simulink model "Quad_PID_FUSION_Close_Loop"  (R2023b)
settings: Solver=ode1  StartTime=0.0  StopTime=400  FixedStep=0.01  RelTol=1e-3
values from neighbouring files (symbols this model uses):
  Quad_Model = struct(     'Ixx', 0.016,      'Iyy', 0.016,      'Izz', 0.0274,      'Im', 3.789e-6,      'mass', 1,      'g', 9.8)    [Quad_PID_FUSION_Pipeline.m]    (also in Quad_PID_FUSION_Pipeline_Close_Loop_Attack.m; Quad_PID_FUSION_Pipeline_Close_Loop_Attack_Pipeline.m; Quad_PID_FUSION_Pipeline_Close_Loop_Attack_Pipeline_Reach.m; Quad_PID_FUSION_Pipeline_Close_Loop_Attack_Pipeline_Repeat_V5.m)
  s_x_0 = 0.0    (= 0)    [Quad_PID_FUSION_Pipeline.m]    (also in Quad_PID_FUSION_Pipeline_Loop_Attack_Execution.m = current_norm * cos(angle))
  s_y_0 = 0.0    (= 0)    [Quad_PID_FUSION_Pipeline.m]    (also in Quad_PID_FUSION_Pipeline_Loop_Attack_Execution.m = current_norm * sin(angle))
undefined symbols (not defined in the file or in its folder): DiscIntNeverNeededParam
libraries: simulink x9, rllib x1
(part 1 of 2)
settings Model: SimulationMode=accelerator  Creator=Qi  LastModifiedBy=32977
settings SolverCC: AlgebraicLoopSolver=TrustRegion
settings DataIOCC: ReturnWorkspaceOutputs=off
settings DebuggingCC: UnconnectedInputMsg=warning  UnconnectedOutputMsg=warning  UnconnectedLineMsg=warning  ArithmeticOperatorsInVariantConditions=warning
settings ModelReferenceCC: EnableRefExpFcnMdlSchedulingChecks=on
settings SFSimCC: CustomCodeUndefinedFunction=UseInterfaceOnly

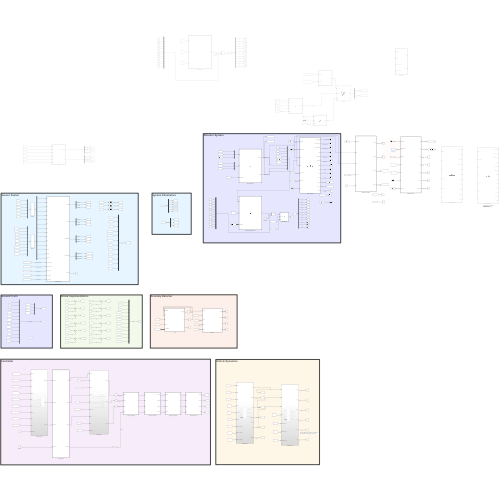
[thumbnail: Simulink's stored preview of the top-level diagram]
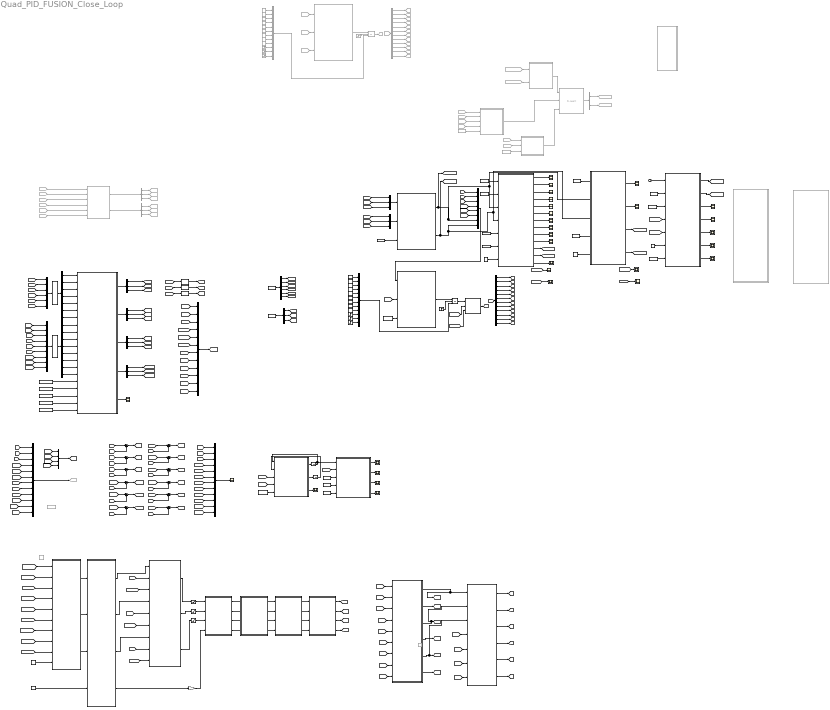
== system Quad_PID_FUSION_Close_Loop ==
  note: Fix the problem of non-covergence at small spoofing distance by adaptive PID tuning
  note: Attacker System
  note: System Parameters
  note: Anomaly Detector
  note: Sensor Fusion
  note: Vehicle Dynamics
  note: Controller
  note: Ground Truth
  note: Attack Implementation
  note: The initial condition of the integrator here is changed to 10,
      | so the intial position of drone is going to be [0,0,10]
  Attack Dynamics : MATLAB Function  Commented=on  TreatAsAtomicUnit=on
  Attack Injection : MATLAB Function  TreatAsAtomicUnit=on
  Attack Time : Step  Time=0  SampleTime=0
  Attacker Observation : MATLAB Function  TreatAsAtomicUnit=on
  Attacker Redirection MPC : MATLAB Function  TreatAsAtomicUnit=on
  Attacker redirection : MATLAB Function  TreatAsAtomicUnit=on
  Attacker redirection1 : MATLAB Function  Commented=on  TreatAsAtomicUnit=on
  Attacker redirection2 : MATLAB Function  Commented=on  TreatAsAtomicUnit=on
  Attacker redirection3 : MATLAB Function  TreatAsAtomicUnit=on
  Attitude Controller : Subsystem
  Attitude Dynamics : Subsystem
  Clock : Clock
  Constant : Constant  Commented=on  Value=10
  Constant{1..2,13..19} (9 alike) : Constant  Value=0
  Constant{4..12} (9 alike) : Constant  Commented=on  Value=0
  Constant20 : Constant  Value=Quad_Model  OutDataTypeStr=Bus: Quad_Model_Bus
  Constant21 : Constant  Value=Quad_Model  OutDataTypeStr=Bus: Quad_Model_Bus
  Constant22 : Constant  Value=0.01
  Constant23 : Constant  Value=0.01
  Constant24 : Constant  Value=0.01
  Constant3 : Constant  Value=0.5
  Demux : Demux  Outputs=9
  Demux1 : Demux  Commented=on  Outputs=3
  Demux{2,4..6,10} (5 alike) : Demux  Outputs=3
  Demux11 : Demux  Outputs=12
  Demux12 : Demux  Commented=on  Outputs=2
  Demux3 : Demux  Commented=on  Outputs=3
  Demux7 : Demux  Commented=on  Outputs=12
  Demux8 : Demux  Outputs=6
  Demux9 : Demux  Outputs=6
  Detector : MATLAB Function  TreatAsAtomicUnit=on
  Discrete Derivative3 : simulink/Discrete/Discrete Derivative  gainval=1.0  ICPrevScaledInput=0.0  OutMin=[]  OutMax=[]  OutDataType=fixdt(1, 16)  OutScaling=2^-10  DoSatur=off
  Discrete Derivative4 : simulink/Discrete/Discrete Derivative  gainval=1.0  ICPrevScaledInput=0.0  OutMin=[]  OutMax=[]  OutDataType=fixdt(1, 16)  OutScaling=2^-10  DoSatur=off
  Discrete Derivative5 : simulink/Discrete/Discrete Derivative  gainval=1.0  ICPrevScaledInput=0.0  OutMin=[]  OutMax=[]  OutDataType=fixdt(1, 16)  OutScaling=2^-10  DoSatur=off
  EKF : MATLAB Function  TreatAsAtomicUnit=on
  From Workspace1 : FromWorkspace  VariableName=System_Noise
  From Workspace10 : FromWorkspace  VariableName=WaypointSeries
  From Workspace11 : FromWorkspace  Commented=on  VariableName=s_x_0_series
  From Workspace12 : FromWorkspace  VariableName=Attacker_Noise
  From Workspace13 : FromWorkspace  VariableName=Spoofing_Target
  From Workspace14 : FromWorkspace  VariableName=S_Norm
  From Workspace15 : FromWorkspace  VariableName=Delta_S_Lim
  From Workspace16 : FromWorkspace  VariableName=Spoofing_Target
  From Workspace17 : FromWorkspace  VariableName=Spoofing_Target
  From Workspace18 : FromWorkspace  VariableName=Delta_S_Lim
  From Workspace19 : FromWorkspace  Commented=on  VariableName=Spoofing_Target
  From Workspace2 : FromWorkspace  VariableName=GPS_Position_Noise
  From Workspace20 : FromWorkspace  Commented=on  VariableName=Spoofing_Target
  From Workspace21 : FromWorkspace  VariableName=Target_R
  From Workspace22 : FromWorkspace  VariableName=Delta_S_Lim
  From Workspace23 : FromWorkspace  VariableName=Attack_Start_T
  From Workspace3 : FromWorkspace  VariableName=GPS_Velocity_Noise
  From Workspace4 : FromWorkspace  VariableName=IMU_Acc_Noise
  From Workspace5 : FromWorkspace  VariableName=IMU_Gyro_Noise
  From Workspace6 : FromWorkspace  VariableName=IMU_Mag_Noise
  From Workspace7 : FromWorkspace  VariableName=Gamma
  From Workspace8 : FromWorkspace  VariableName=Delta_1
  From Workspace9 : FromWorkspace  VariableName=Delta_2
  From102 : From  Commented=on  GotoTag=pos_y_diff
  From103 : From  Commented=on  GotoTag=pos_z_diff
  From142 : From  Commented=on  GotoTag=vel_y
  From143 : From  Commented=on  GotoTag=pos_x
  From144 : From  Commented=on  GotoTag=pos_x
  From145 : From  Commented=on  GotoTag=pos_y
  From146 : From  Commented=on  GotoTag=pos_y
  From147 : From  Commented=on  GotoTag=vel_x
  From150 : From  Commented=on  GotoTag=attacker_pos_obs
  From151 : From  Commented=on  GotoTag=attacker_vel_obs
  From16 : From  Commented=on  GotoTag=pos_x_diff
  From20 : From  Commented=on  GotoTag=vel_y_diff
  From21 : From  Commented=on  GotoTag=vel_z_diff
  From49 : From  Commented=on  GotoTag=input
  From50 : From  Commented=on  GotoTag=X
  From51 : From  Commented=on  GotoTag=s
  From52 : From  Commented=on  GotoTag=s
  From56 : From  Commented=on  GotoTag=vel_x_diff
  GPS : MATLAB Function  Commented=on  TreatAsAtomicUnit=on
  GPS Sensor : MATLAB Function  Commented=on  TreatAsAtomicUnit=on
  GPS Spoofing Attack Dynamics : MATLAB Function  TreatAsAtomicUnit=on
  GPS ZOH : ZeroOrderHold  SampleTime=0.1
  GPSIMUFUSION : MATLAB Function  TreatAsAtomicUnit=on
  Gain1 : Gain  Gain=20
  Goto12 : Goto  Commented=on  GotoTag=pos_x_gps
  Goto13 : Goto  Commented=on  GotoTag=pos_y_gps
  Goto14 : Goto  Commented=on  GotoTag=pos_z_gps
  Goto15 : Goto  Commented=on  GotoTag=vel_x_gps
  Goto16 : Goto  Commented=on  GotoTag=vel_y_gps
  Goto17 : Goto  Commented=on  GotoTag=vel_z_gps
  Goto24 : Goto  Commented=on  GotoTag=s
  Goto25 : Goto  Commented=on  GotoTag=s_1
  Goto26 : Goto  Commented=on  GotoTag=s_2
  Goto27 : Goto  Commented=on  GotoTag=s_3
  Goto28 : Goto  Commented=on  GotoTag=s_4
  Goto41 : Goto  Commented=on  GotoTag=s_5
  Goto42 : Goto  Commented=on  GotoTag=s_6
  Goto43 : Goto  Commented=on  GotoTag=s_7
  Goto44 : Goto  Commented=on  GotoTag=s_8
  Goto45 : Goto  Commented=on  GotoTag=s_9
  Goto46 : Goto  Commented=on  GotoTag=s_10
  Goto47 : Goto  Commented=on  GotoTag=s_11
  Goto48 : Goto  Commented=on  GotoTag=s_12
  Goto54 : Goto  Commented=on  GotoTag=X
  Goto91 : Goto  Commented=on  GotoTag=new_s_vx_rl
  Goto92 : Goto  Commented=on  GotoTag=new_s_vy_rl
  IMU ZOH : ZeroOrderHold  SampleTime=0.01
  Integrator1 : Integrator  InitialCondition=1*[0,0,0,0,0,0,0,0,10,0,0,0]
  Integrator100 : Integrator  Commented=on  ExternalReset=rising  InitialConditionSource=external  InitialCondition=0.002*[1,0,0,0,0,0,0,0,0,0,0,0]
  Integrator2 : Integrator  InitialCondition=0*eye(12)
  Integrator4 : Integrator  ExternalReset=rising  InitialConditionSource=external  InitialCondition=0.002*[1,0,0,0,0,0,0,0,0,0,0,0]
  MATLAB Function : MATLAB Function  Commented=on  TreatAsAtomicUnit=on
  MATLAB Function1 : MATLAB Function  Commented=on  TreatAsAtomicUnit=on
  MATLAB Function2 : MATLAB Function  Commented=on  TreatAsAtomicUnit=on
  Mux : Mux
  Mux{1..2,6..7} (4 alike) : Mux  Inputs=12
  Mux10 : Mux  Inputs=8
  Mux3 : Mux  Inputs=9
  Mux4 : Mux  Inputs=6
  Mux5 : Mux  Commented=on  Inputs=12
  Mux8 : Mux  Inputs=3
  Mux9 : Mux  Inputs=3
  Position Controller : Subsystem
  Position Dynamics : Subsystem
  RLSpoofer : rllib/RL Agent  Commented=on  Agent=agent  ExternalActionAsInput=off  ProvideLastAction=off  ProvideCumRwd=off  TreatAsDirectFeedthrough=on  UseStrictObservationDataTypes=off
  Saturation : Saturate  UpperLimit=1  LowerLimit=-1
  Saturation1 : Saturate  UpperLimit=1  LowerLimit=-1
  Saturation2 : Saturate  UpperLimit=1  LowerLimit=-1
  Scope{,1..28} (29 alike) : Scope
  Step1 : Step  Commented=on  Time=0  After=s_y_0  SampleTime=0
  Step2 : Step  Commented=on  Time=0  After=0  SampleTime=0
  Step3 : Step  Commented=on  Time=3  SampleTime=0
  Step4 : Step  Commented=on  Time=0  After=s_x_0  SampleTime=0
  Step5 : Step  Time=0  After=0  SampleTime=0
  Step6 : Step  Time=0  After=0  SampleTime=0
  Step8 : Step  Time=0  After=0  SampleTime=0
  Sum{12..23} (12 alike) : Sum  Inputs=|+-
  Thrust_to_Attitude : MATLAB Function  TreatAsAtomicUnit=on
  "disturbance " : Constant  Commented=on  Value=0
  "motor_speed_to_throttle " : MATLAB Function  TreatAsAtomicUnit=on
  motor_speed_to_thrust : MATLAB Function  TreatAsAtomicUnit=on
  throttle_to_motor_speed : MATLAB Function  TreatAsAtomicUnit=on
  thrust_to_motor_speed : MATLAB Function  TreatAsAtomicUnit=on
  yaw_sp : Constant  Value=0
  wires:
  yaw_sp/1 -> Thrust_to_Attitude/4(yaw_setpoint)
  Thrust_to_Attitude/4(thrust_body) -> Gain1/1
  [pos_x_fused] -> Position Controller/2(pos_x)
  [target_y] -> Position Controller/4(pos_sp_y)
  [pos_z_fused] -> Position Controller/8(pos_z)
  [target_z] -> Position Controller/7(pos_sp_z)
  Position Controller/1(thrust_sp_x) -> Thrust_to_Attitude/1(thrust_enu_x)
  Position Controller/2(thrust_sp_y) -> Thrust_to_Attitude/2(thrust_enu_y)
  Position Controller/3(thrust_sp_z) -> Thrust_to_Attitude/3(thrust_enu_z)
  [yaw_fused] -> Attitude Controller/8(yaw)
  [roll_fused] -> Attitude Controller/2(roll)
  [pitch_fused] -> Attitude Controller/5(pitch)
  Thrust_to_Attitude/1(roll_sp) -> Attitude Controller/1(roll_sp)
  Thrust_to_Attitude/2(pitch_sp) -> Attitude Controller/4(pitch_sp)
  Thrust_to_Attitude/3(yaw_sp) -> Attitude Controller/7(yaw_sp)
  Attitude Controller/2(torque_y) -> Saturation1/1
  Attitude Controller/1(torque_x) -> Saturation/1
  Attitude Controller/3(torque_z) -> Saturation2/1
  [vel_x_fused] -> Position Controller/3(vel_x)
  [pos_y_fused] -> Position Controller/5(pos_y)
  [vel_y_fused] -> Position Controller/6(vel_y)
  [vel_z_fused] -> Position Controller/9(vel_z)
  [roll_rate_fused] -> Attitude Controller/3(roll_rate)
  [pitch_rate_fused] -> Attitude Controller/6(pitch_rate)
  [yaw_rate_fused] -> Attitude Controller/9(yaw_rate)
  Attitude Dynamics/3(pitch) -> Position Dynamics/2(pitch), [pitch]  "pitch"
  Attitude Dynamics/1(roll) -> [roll], Position Dynamics/1(roll)  "roll"
  Attitude Dynamics/5(yaw) -> [yaw], Position Dynamics/3(yaw)  "yaw"
  [roll_rate] -> Attitude Dynamics/4(roll_dot)
  [pitch_rate] -> Attitude Dynamics/5(pitch_dot)
  [yaw_rate] -> Attitude Dynamics/6(yaw_dot)
  Attitude Dynamics/2(roll_rate) -> [roll_rate]  "roll_rate"
  Attitude Dynamics/4(pitch_rate) -> [pitch_rate]  "pitch_rate"
  Attitude Dynamics/6(yaw_rate) -> [yaw_rate]  "yaw_rate"
  Position Dynamics/1(pos_x) -> [pos_x]  "pos_x"
  Position Dynamics/3(pos_y) -> [pos_y]  "pos_y"
  Position Dynamics/4(vel_y) -> [vel_y]  "vel_y"
  Position Dynamics/5(pos_z) -> [pos_z]  "pos_z"
  Position Dynamics/6(vel_z) -> [vel_z]  "vel_z"
  Constant3/1 -> Position Controller/10(Thrust_hover)
  thrust_to_motor_speed/1(w_1) -> "motor_speed_to_throttle "/1(w_1)
  thrust_to_motor_speed/3(w_3) -> "motor_speed_to_throttle "/3(w_3)
  thrust_to_motor_speed/4(w_4) -> "motor_speed_to_throttle "/4(w_4)
  thrust_to_motor_speed/2(w_2) -> "motor_speed_to_throttle "/2(w_2)
  "motor_speed_to_throttle "/1(throttle_1) -> throttle_to_motor_speed/1(throttle_1)
  "motor_speed_to_throttle "/2(throttle_2) -> throttle_to_motor_speed/2(throttle_2)
  "motor_speed_to_throttle "/3(throttle_3) -> throttle_to_motor_speed/3(throttle_3)
  "motor_speed_to_throttle "/4(throttle_4) -> throttle_to_motor_speed/4(throttle_4)
  throttle_to_motor_speed/1(w_1) -> motor_speed_to_thrust/1(w_1)
  throttle_to_motor_speed/2(w_2) -> motor_speed_to_thrust/2(w_2)
  throttle_to_motor_speed/3(w_3) -> motor_speed_to_thrust/3(w_3)
  throttle_to_motor_speed/4(w_4) -> motor_speed_to_thrust/4(w_4)
  Gain1/1 -> thrust_to_motor_speed/4(thrust)  "thrust_sp"
  Position Dynamics/2(vel_x) -> [vel_x]  "vel_x"
  Saturation/1 -> thrust_to_motor_speed/1(torque_x)  "torque_x_sp"
  Saturation1/1 -> thrust_to_motor_speed/2(torque_y)  "torque_y_sp"
  Saturation2/1 -> thrust_to_motor_speed/3(torque_z)  "torque_z_sp"
  Discrete Derivative5/1 -> [acc_z]  "acc_z"
  Discrete Derivative3/1 -> [acc_x]  "acc_x"
  [vel_z_diff] -> Discrete Derivative5/1
  [vel_x_diff] -> Discrete Derivative3/1
  Discrete Derivative4/1 -> [acc_y]  "acc_y"
  [vel_y_diff] -> Discrete Derivative4/1
  GPS/2(vel_gps) -> Demux3/1
  Demux1/1 -> Goto12/1  "pos_x_gps"
  Demux1/2 -> Goto13/1  "pos_y_gps"
  Demux1/3 -> Goto14/1  "pos_z_gps"
  Demux3/1 -> Goto15/1  "vel_x_gps"
  Demux3/3 -> Goto17/1  "vel_z_gps"
  Demux3/2 -> Goto16/1  "vel_y_gps"
  Demux4/2 -> [pos_y_fused]  "pos_y_fused"
  Demux4/1 -> [pos_x_fused]  "pos_x_fused"
  GPSIMUFUSION/1(fusedPos) -> Demux4/1
  Demux4/3 -> [pos_z_fused]  "pos_z_fused"
  Demux5/3 -> [yaw_fused]  "yaw_fused"
  Demux5/1 -> [roll_fused]  "roll_fused"
  Demux5/2 -> [pitch_fused]  "pitch_fused"
  GPSIMUFUSION/3(fusedOrientEuler) -> Demux5/1
  Mux3/1 -> IMU ZOH/1
  IMU ZOH/1 -> Demux/1
  [roll_diff] -> Mux3/4
  [pitch_diff] -> Mux3/5
  [yaw_diff] -> Mux3/6
  Demux/9 -> GPSIMUFUSION/15(yaw_rate)
  Demux/8 -> GPSIMUFUSION/14(pitch_rate)
  Demux/7 -> GPSIMUFUSION/13(roll_rate)
  Demux/6 -> GPSIMUFUSION/12(yaw)
  Demux/5 -> GPSIMUFUSION/11(pitch)
  Demux/4 -> GPSIMUFUSION/10(roll)
  Demux/3 -> GPSIMUFUSION/9(acc_z)
  Demux/2 -> GPSIMUFUSION/8(acc_y)
  Demux/1 -> GPSIMUFUSION/7(acc_x)
  Demux9/1 -> GPSIMUFUSION/1(pos_x)
  Demux9/2 -> GPSIMUFUSION/2(pos_y)
  Demux9/3 -> GPSIMUFUSION/3(pos_z)
  Demux9/4 -> GPSIMUFUSION/4(vel_x)
  Demux9/5 -> GPSIMUFUSION/5(vel_y)
  Demux9/6 -> GPSIMUFUSION/6(vel_z)
  GPS ZOH/1 -> Demux9/1
  GPS/1(local_pos_gps) -> Demux1/1
  [vel_x] -> Sum23/1
  [pos_x_diff] -> Mux2/7
  Sum12/1 -> [roll_rate_diff]
  Sum13/1 -> [pitch_rate_diff]
  Sum16/1 -> [pitch_diff]
  [pitch_rate] -> Sum13/1
  [vel_x_diff] -> Mux2/10
  [roll_diff] -> Mux2/1
  [yaw_diff] -> Mux2/3
  Sum17/1 -> [yaw_diff]
  [s_10] -> Sum23/2  "s10"
  [s_9] -> Sum21/2  "s9"
  [pos_z] -> Sum21/1
  [s_5] -> Sum13/2  "s5"
  [s_11] -> Sum19/2  "s11"
  [s_7] -> Sum18/2  "s7"
  [vel_y_diff] -> Mux2/11
  [roll] -> Sum15/1
  Mux2/1 -> Scope3/1  "x_diff"
  [pos_x] -> Sum18/1
  [pos_y] -> Sum20/1
  [yaw_rate] -> Sum14/1
  Sum14/1 -> [yaw_rate_diff]
  [vel_z] -> Sum22/1
  [roll_rate] -> Sum12/1
  Sum21/1 -> [pos_z_diff]
  [s_6] -> Sum14/2  "s6"
  [vel_z_diff] -> Mux2/12
  [pitch] -> Sum16/1
  [pos_z_diff] -> Mux2/9
  Sum22/1 -> [vel_z_diff]
  [pitch_diff] -> Mux2/2
  [s_1] -> Sum15/2  "s1"
  [s_4] -> Sum12/2  "s4"
  [roll_rate_diff] -> Mux2/4
  [pitch_rate_diff] -> Mux2/5
  [s_2] -> Sum16/2  "s2"
  [s_12] -> Sum22/2  "s12"
  [vel_y] -> Sum19/1
  [yaw] -> Sum17/1
  Sum15/1 -> [roll_diff]
  Sum23/1 -> [vel_x_diff]
  [yaw_rate_diff] -> Mux2/6
  Sum20/1 -> [pos_y_diff]
  Sum18/1 -> [pos_x_diff]
  Sum19/1 -> [vel_y_diff]
  [s_3] -> Sum17/2  "s3"
  [s_8] -> Sum20/2  "s8"
  [pos_y_diff] -> Mux2/8
  Demux7/12 -> Goto48/1  "s_12"
  From49/1 -> Attack Dynamics/2(input)
  Demux7/11 -> Goto47/1  "s_11"
  Demux7/1 -> Goto25/1  "s_1"
  From51/1 -> Attack Dynamics/3(s)
  From52/1 -> Demux7/1
  Demux7/4 -> Goto28/1  "s_4"
  Demux7/3 -> Goto27/1  "s_3"
  Integrator100/1 -> Goto24/1
  Demux7/6 -> Goto42/1  "s_6"
  Demux7/5 -> Goto41/1  "s_5"
  From50/1 -> Attack Dynamics/1(X)
  Demux7/10 -> Goto46/1  "s_10"
  Demux7/2 -> Goto26/1  "s_2"
  Attack Dynamics/1(s_d) -> Integrator100/1
  Constant7/1 -> Mux5/4
  Constant8/1 -> Mux5/2
  Constant12/1 -> Mux5/9
  Constant5/1 -> Mux5/7
  Constant6/1 -> Mux5/5
  Step2/1 -> Mux5/12
  Step1/1 -> Mux5/11
  Constant10/1 -> Mux5/8
  Mux5/1 -> Integrator100/3
  Constant11/1 -> Mux5/1
  Constant9/1 -> Mux5/6
  Constant4/1 -> Mux5/3
  [pos_x] -> Mux6/7
  [yaw_rate] -> Mux6/6
  [vel_y] -> Mux6/11
  [pitch_rate] -> Mux6/5
  [roll_rate] -> Mux6/4
  [roll] -> Mux6/1
  [thrust] -> Mux/4
  [torque_x] -> Mux/1
  [torque_y] -> Mux/2
  Mux/1 -> [input]
  [yaw] -> Mux6/3
  [vel_x] -> Mux6/10
  [pos_y] -> Mux6/8
  Mux6/1 -> Goto54/1  "x_ground_truth"
  [torque_z] -> Mux/3
  [vel_z] -> Mux6/12
  [pos_z] -> Mux6/9
  [pitch] -> Mux6/2
  motor_speed_to_thrust/4(thrust) -> [thrust]
  motor_speed_to_thrust/2(torque_y) -> [torque_y]
  motor_speed_to_thrust/1(torque_x) -> [torque_x]
  motor_speed_to_thrust/3(torque_z) -> [torque_z]
  [torque_x] -> Attitude Dynamics/1(torque_x)
  [torque_y] -> Attitude Dynamics/2(torque_y)
  [torque_z] -> Attitude Dynamics/3(torque_z)
  [thrust] -> Position Dynamics/4(thrust)
  Step3/1 -> Integrator100/2
  From16/1 -> GPS/1(pos_x)
  From102/1 -> GPS/2(pos_y)
  From103/1 -> GPS/3(pos_z)
  GPSIMUFUSION/4(fusedAngularVel) -> Demux2/1
  Demux2/2 -> [pitch_rate_fused]  "pitch_rate_fused"
  Demux2/3 -> [yaw_rate_fused]  "yaw_rate_fused"
  Demux2/1 -> [roll_rate_fused]  "roll_rate_fused"
  GPSIMUFUSION/2(fusedVel) -> Demux6/1
  Demux6/1 -> [vel_x_fused]  "vel_x_fused"
  Demux6/2 -> [vel_y_fused]  "vel_y_fused"
  Demux6/3 -> [vel_z_fused]  "vel_z_fused"
  From56/1 -> GPS/4(vel_x)
  From20/1 -> GPS/5(vel_y)
  From21/1 -> GPS/6(vel_z)
  Demux7/7 -> Goto43/1  "s_7"
  Demux7/8 -> Goto44/1  "s_8"
  Demux7/9 -> Goto45/1  "s_9"
  Mux1/1 -> [x_hat]  "x_hat"
  EKF/2(P_d) -> Integrator2/1
  Integrator2/1 -> EKF/2(P)
  EKF/1(x_hat_d_ekf) -> Integrator1/1
  Integrator1/1 -> EKF/1(x_hat_ekf), Detector/1(x_hat_ekf)  "x_hat_ekf"
  [input] -> EKF/4(input)
  EKF/3(k) -> Scope1/1
  [x_hat] -> Detector/2(Y)
  Detector/4(S_out) -> Scope5/1  "S_out"
  Detector/2(c_alarm) -> Scope12/1  "c_alarm"
  Detector/1(r_alarm) -> Scope9/1  "r_alarm"
  Detector/3(r) -> Scope2/1  "r"
  [yaw_rate_fused] -> Mux1/6
  [pitch_rate_fused] -> Mux1/5
  [roll_rate_fused] -> Mux1/4
  [yaw_fused] -> Mux1/3
  [pitch_fused] -> Mux1/2
  [roll_fused] -> Mux1/1
  [vel_z_fused] -> Mux1/12
  [vel_y_fused] -> Mux1/11
  [vel_x_fused] -> Mux1/10
  [pos_z_fused] -> Mux1/9
  [pos_y_fused] -> Mux1/8
  [pos_x_fused] -> Mux1/7
  [x_hat] -> EKF/3(Y)
  From Workspace1/1 -> Demux8/1
  Demux8/1 -> [Noise_1]
  Demux8/2 -> [Noise_2]
  Demux8/3 -> [Noise_3]
  Demux8/4 -> [Noise_4]
  Demux8/5 -> [Noise_5]
  Demux8/6 -> [Noise_6]
  [Noise_1] -> Attitude Dynamics/7(disturbance_torque_x)
  [Noise_2] -> Attitude Dynamics/8(disturbance_torque_y)
  [Noise_3] -> Attitude Dynamics/9(disturbance_torque_z)
  [Noise_4] -> Position Dynamics/5(disturbance_force_x)
  [Noise_5] -> Position Dynamics/6(disturbance_force_y)
  [Noise_6] -> Position Dynamics/7(disturbance_force_z)
  Mux4/1 -> GPS ZOH/1
  [acc_x] -> Mux3/1
  [acc_y] -> Mux3/2
  [acc_z] -> Mux3/3
  [yaw_rate_diff] -> Mux3/9
  [pitch_rate_diff] -> Mux3/8
  [roll_rate_diff] -> Mux3/7
  From Workspace4/1 -> GPSIMUFUSION/18(imu_acc_noise)  "imu_acc_noise"
  From Workspace5/1 -> GPSIMUFUSION/19(imu_gyro_noise)  "imu_gyro_noise"
  From Workspace6/1 -> GPSIMUFUSION/20(imu_mag_noise)  "imu_mag_noise"
  From Workspace2/1 -> GPSIMUFUSION/16(gps_position_noise)  "gps_position_noise"
  From Workspace3/1 -> GPSIMUFUSION/17(gps_velocity_noise)  "gps_velocity_noise"
  [vel_y_diff] -> Mux4/5
  [vel_x_diff] -> Mux4/4
  [vel_z_diff] -> Mux4/6
  [pos_x_diff] -> Mux4/1
  [pos_z_diff] -> Mux4/3
  [pos_y_diff] -> Mux4/2
  From Workspace7/1 -> Detector/3(gamma)  "gamma"
  From Workspace8/1 -> Detector/4(delta_1)  "delta_1"
  From Workspace9/1 -> Detector/5(delta_2)  "delta_2"
  From Workspace10/1 -> Demux10/1  "waypoints"
  Demux10/1 -> [target_x]
  Demux10/2 -> [target_y]
  Demux10/3 -> [target_z]
  [target_x] -> Position Controller/1(pos_sp_x)
  GPSIMUFUSION/5(imu_counter) -> Scope/1
  Step4/1 -> Mux5/10
  Attack Time/1 -> Integrator4/2
  GPS Spoofing Attack Dynamics/1(s_d) -> Integrator4/1
  Demux11/2 -> [s_2]  "s_2"
  Constant1/1 -> Mux7/8
  Demux11/9 -> [s_9]  "s_9"
  Mux7/1 -> Integrator4/3
  Constant13/1 -> Mux7/9
  Integrator4/1 -> Attack Injection/1("s ")
  Demux11/8 -> [s_8]  "s_8"
  Demux11/7 -> [s_7]  "s_7"
  Constant15/1 -> Mux7/7
  Constant19/1 -> Mux7/6
  Constant14/1 -> Mux7/3
  Demux11/1 -> [s_1]  "s_1"
  Step6/1 -> Mux7/12
  Constant2/1 -> Mux7/1
  Demux11/6 -> [s_6]  "s_6"
  Constant18/1 -> Mux7/2
  Demux11/11 -> [s_11]  "s_11"
  Demux11/5 -> [s_5]  "s_5"
  Demux11/3 -> [s_3]  "s_3"
  Demux11/4 -> [s_4]  "s_4"
  Constant16/1 -> Mux7/5
  [s] -> Demux11/1
  Constant17/1 -> Mux7/4
  Demux11/12 -> [s_12]  "s_12"
  [s] -> GPS Spoofing Attack Dynamics/2(s)
  Demux11/10 -> [s_10]  "s_10"
  Constant20/1 -> GPS Spoofing Attack Dynamics/3(Quad_Model)
  Constant21/1 -> EKF/5(Quad_Model)
  [vel_z] -> Mux8/3
  [pos_y] -> Mux9/2
  [pos_z] -> Mux9/3
  [pos_x] -> Mux9/1
  [vel_x] -> Mux8/1
  [vel_y] -> Mux8/2
  Mux8/1 -> Attacker Observation/2(vel)
  Mux9/1 -> Attacker Observation/1(pos)
  [pitch] -> Mux10/2
  [roll] -> Mux10/1
  [roll_rate] -> Mux10/4
  [pitch_rate] -> Mux10/5
  [yaw_rate] -> Mux10/6
  [yaw] -> Mux10/3
  Attacker Observation/1(victim_pos) -> [attacker_pos_obs], Attacker redirection/3(pos), Attacker Redirection MPC/2(pos), Mux10/7  "attacker_pos_obs"
  Attacker Observation/2(victim_vel) -> [attacker_vel_obs], Mux10/8, Attacker Redirection MPC/3(vel), Attacker redirection/4(vel)  "attacker_vel_obs"
  Mux10/1 -> GPS Spoofing Attack Dynamics/1(X)
  From Workspace12/1 -> Attacker Observation/3(attacker_noise)
  From Workspace14/1 -> Attacker redirection/5(s_norm_lim)  "s_norm_lim"
  From Workspace13/1 -> Attacker redirection/1(target_pos)  "target_pos"
  Attacker redirection/11(new_s_vx) -> [new_s_vx]  "new_s_vx"
  Attacker redirection/12(new_s_vy) -> [new_s_vy]  "new_s_vy"
  Step8/1 -> Mux7/10
  Step5/1 -> Mux7/11
  Attack Injection/1(s) -> [s]
  [new_s_vx_pid] -> Attack Injection/2(new_vx)
  [new_s_vy_pid] -> Attack Injection/3(new_vy)
  Attacker redirection/9(error_x) -> Scope8/1  "error_x"
  Attacker redirection/1(p_control_angle) -> Scope11/1  "p_control_angle"
  Attacker redirection/6(direction_diff) -> Scope13/1  "direction_diff"
  Attacker redirection/4(theta) -> Scope14/1  "theta"
  Attacker redirection/5(current_theta) -> Scope15/1  "current_theta"
  Attacker redirection/10(error_y) -> Scope4/1  "error_y"
  Constant23/1 -> Attacker redirection/7(dt)
  Attacker redirection/7(gamma) -> Scope6/1
  Attacker redirection/13(delta_s) -> Scope7/1  "delta_s"
  Attacker redirection/8(beta) -> Scope10/1  "beta"
  From Workspace15/1 -> Attacker redirection/6(delta_s_lim)  "delta_s_lim"
  From Workspace16/1 -> Attacker Redirection MPC/1(target_pos)
  From Workspace18/1 -> Attacker Redirection MPC/4(a_s_lim)  "delta_s_lim"
  Constant22/1 -> Attacker Redirection MPC/5(dt)
  Attacker Redirection MPC/4(new_s_vy) -> [new_s_vy_mpc]  "new_s_vy_mpc"
  Attacker Redirection MPC/3(new_s_vx) -> [new_s_vx_mpc]  "new_s_vx_mpc"
  Attacker Redirection MPC/2(a_s_opt_y) -> Scope18/1  "a_s_opt_y"
  Attacker Redirection MPC/1(a_s_opt_x) -> Scope24/1  "a_s_opt_x"
  [new_s_vx_mpc] -> Scope16/1
  [new_s_vy_mpc] -> Scope17/1
  From145/1 -> MATLAB Function/2(pos_y)
  From144/1 -> MATLAB Function/1(pos_x)
  From147/1 -> MATLAB Function/3(vel_x)
  From142/1 -> MATLAB Function/4(vel_y)
  From Workspace19/1 -> MATLAB Function/5(target)  "target_pos"
  MATLAB Function/1(reward) -> RLSpoofer/2  "rl_reward"
  From146/1 -> MATLAB Function1/2(pos_y)
  From143/1 -> MATLAB Function1/1(pos_x)
  From Workspace20/1 -> MATLAB Function1/3(target)  "target_pos"
  MATLAB Function1/1(is_done) -> RLSpoofer/3  "rl_done"
  RLSpoofer/1 -> Demux12/1
  Demux12/1 -> Goto91/1  "new_s_vx_rl"
  Demux12/2 -> Goto92/1  "new_s_vy_rl"
  From150/1 -> MATLAB Function2/1(attacker_pos)
  From151/1 -> MATLAB Function2/2(attacker_vel)
  MATLAB Function2/1(obs) -> RLSpoofer/1  "rl_obs"
  Attacker redirection/2(p_control_position_x) -> Scope25/1  "p_control_position_x"
  Attacker redirection/3(p_control_position_y) -> Scope26/1  "p_control_position_y"
  From Workspace21/1 -> Attacker redirection/2(target_radius)  "target_radius"
  From Workspace17/1 -> Attacker redirection3/3(target_pos)
  [attacker_pos_obs] -> Attacker redirection3/4(pos)
  [attacker_vel_obs] -> Attacker redirection3/5(vel)
  Constant24/1 -> Attacker redirection3/6(dt)
  From Workspace22/1 -> Attacker redirection3/7(delta_s_lim)  "delta_s_lim"
  Attacker redirection3/1(s_vx) -> [new_s_vx_pid]  "new_s_vx_pid"
  Attacker redirection3/2(s_vy) -> [new_s_vy_pid]  "new_s_vy_pid"
  Attacker redirection3/3(a_sx) -> Scope19/1  "a_sx_pid"
  Attacker redirection3/4(a_sy) -> Scope20/1  "a_sy_pid"
  Attacker redirection3/5(v_ref_x) -> Scope21/1  "v_ref_x_pid"
  Attacker redirection3/6(v_ref_y) -> Scope22/1  "v_ref_y_pid"
  Attacker redirection3/7(delta_s_pid) -> Scope23/1  "delta_s_pid"
  [new_s_vy] -> Scope28/1
  [new_s_vx] -> Scope27/1
  Clock/1 -> Attacker redirection3/1(current_time)  "current_time"
  From Workspace23/1 -> Attacker redirection3/2(attack_start_time)  "delta_s_lim"

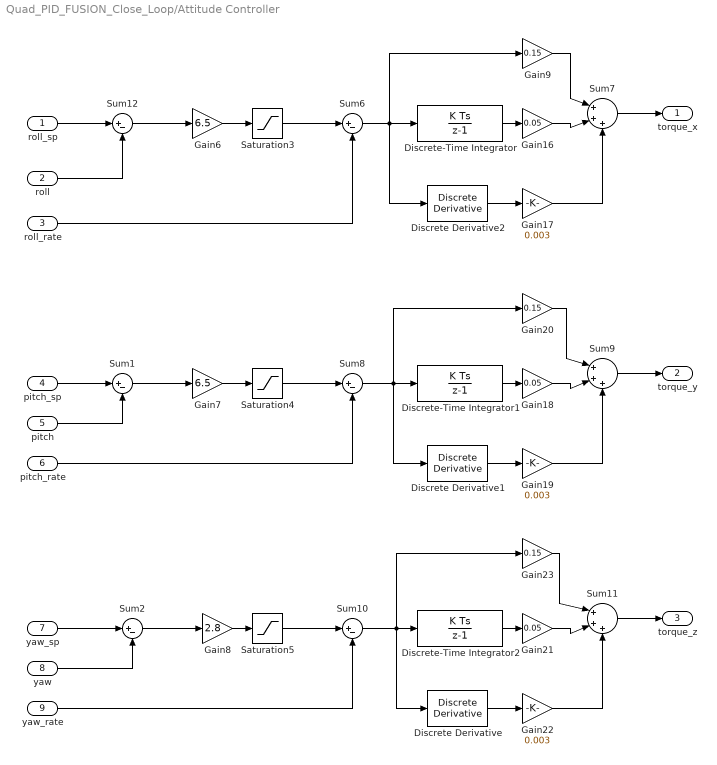
== system Quad_PID_FUSION_Close_Loop/Attitude Controller ==
  roll_sp : Inport
  roll : Inport  Port=2
  roll_rate : Inport  Port=3
  pitch_sp : Inport  Port=4
  pitch : Inport  Port=5
  pitch_rate : Inport  Port=6
  yaw_sp : Inport  Port=7
  yaw : Inport  Port=8
  yaw_rate : Inport  Port=9
  Discrete Derivative : simulink/Discrete/Discrete Derivative  gainval=1.0  ICPrevScaledInput=0.0  OutMin=[]  OutMax=[]  OutDataType=fixdt(1, 16)  OutScaling=2^-10  DoSatur=off
  Discrete Derivative1 : simulink/Discrete/Discrete Derivative  gainval=1.0  ICPrevScaledInput=0.0  OutMin=[]  OutMax=[]  OutDataType=fixdt(1, 16)  OutScaling=2^-10  DoSatur=off
  Discrete Derivative2 : simulink/Discrete/Discrete Derivative  gainval=1.0  ICPrevScaledInput=0.0  OutMin=[]  OutMax=[]  OutDataType=fixdt(1, 16)  OutScaling=2^-10  DoSatur=off
  Discrete-Time Integrator : DiscreteIntegrator  SampleTime=-1  LimitOutput=on  UpperSaturationLimit=0.3  LowerSaturationLimit=-0.3  ICPrevOutput=DiscIntNeverNeededParam  ICPrevScaledInput=DiscIntNeverNeededParam
  Discrete-Time Integrator1 : DiscreteIntegrator  SampleTime=-1  LimitOutput=on  UpperSaturationLimit=0.3  LowerSaturationLimit=-0.3  ICPrevOutput=DiscIntNeverNeededParam  ICPrevScaledInput=DiscIntNeverNeededParam
  Discrete-Time Integrator2 : DiscreteIntegrator  SampleTime=-1  LimitOutput=on  UpperSaturationLimit=0.3  LowerSaturationLimit=-0.3  ICPrevOutput=DiscIntNeverNeededParam  ICPrevScaledInput=DiscIntNeverNeededParam
  Gain16 : Gain  Gain=0.05
  Gain17 : Gain  Gain=0.003
  Gain18 : Gain  Gain=0.05
  Gain19 : Gain  Gain=0.003
  Gain20 : Gain  Gain=0.15
  Gain21 : Gain  Gain=0.05
  Gain22 : Gain  Gain=0.003
  Gain23 : Gain  Gain=0.15
  Gain6 : Gain  Gain=6.5
  Gain7 : Gain  Gain=6.5
  Gain8 : Gain  Gain=2.8
  Gain9 : Gain  Gain=0.15
  Saturation3 : Saturate  UpperLimit=220/180*pi  LowerLimit=-220/180*pi
  Saturation4 : Saturate  UpperLimit=220/180*pi  LowerLimit=-220/180*pi
  Saturation5 : Saturate  UpperLimit=220/180*pi  LowerLimit=-220/180*pi
  Sum{1..2,6,8,10,12} (6 alike) : Sum  Inputs=|+-
  Sum11 : Sum  Inputs=|+++
  Sum7 : Sum  Inputs=|+++
  Sum9 : Sum  Inputs=|+++
  torque_x : Outport  VectorParamsAs1DForOutWhenUnconnected=off
  torque_y : Outport  Port=2  VectorParamsAs1DForOutWhenUnconnected=off
  torque_z : Outport  Port=3  VectorParamsAs1DForOutWhenUnconnected=off
  wires:
  Gain8/1 -> Saturation5/1
  Sum10/1 -> Discrete-Time Integrator2/1, Discrete Derivative/1, Gain23/1
  Sum6/1 -> Discrete-Time Integrator/1, Discrete Derivative2/1, Gain9/1
  Saturation4/1 -> Sum8/1
  Sum7/1 -> torque_x/1
  Discrete-Time Integrator2/1 -> Gain21/1
  Gain16/1 -> Sum7/2
  Sum8/1 -> Discrete-Time Integrator1/1, Discrete Derivative1/1, Gain20/1
  yaw_rate/1 -> Sum10/2
  Saturation5/1 -> Sum10/1
  Gain23/1 -> Sum11/1
  Saturation3/1 -> Sum6/1
  Discrete Derivative1/1 -> Gain19/1
  Gain17/1 -> Sum7/3
  Gain19/1 -> Sum9/3
  Gain22/1 -> Sum11/3
  Discrete Derivative/1 -> Gain22/1
  Gain7/1 -> Saturation4/1
  Discrete-Time Integrator1/1 -> Gain18/1
  Gain18/1 -> Sum9/2
  Gain9/1 -> Sum7/1
  Gain20/1 -> Sum9/1
  Discrete-Time Integrator/1 -> Gain16/1
  roll_rate/1 -> Sum6/2
  Sum9/1 -> torque_y/1
  Discrete Derivative2/1 -> Gain17/1
  Gain21/1 -> Sum11/2
  Gain6/1 -> Saturation3/1
  Sum11/1 -> torque_z/1
  pitch_rate/1 -> Sum8/2
  yaw/1 -> Sum2/2
  Sum1/1 -> Gain7/1
  roll_sp/1 -> Sum12/1
  pitch/1 -> Sum1/2
  Sum2/1 -> Gain8/1
  pitch_sp/1 -> Sum1/1
  roll/1 -> Sum12/2
  yaw_sp/1 -> Sum2/1
  Sum12/1 -> Gain6/1

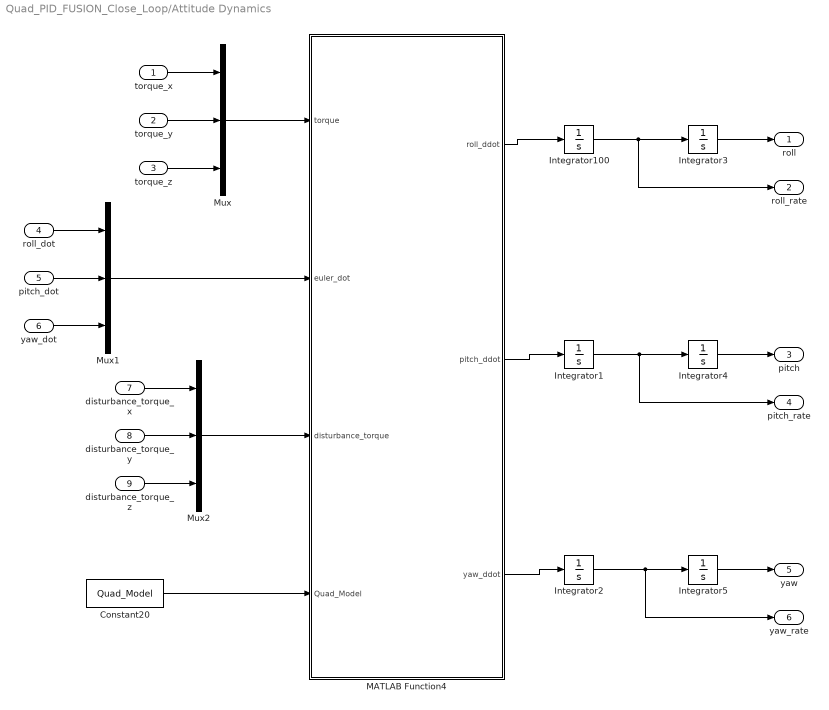
== system Quad_PID_FUSION_Close_Loop/Attitude Dynamics ==
  torque_x : Inport
  torque_y : Inport  Port=2
  torque_z : Inport  Port=3
  roll_dot : Inport  Port=4
  pitch_dot : Inport  Port=5
  yaw_dot : Inport  Port=6
  disturbance_torque_x : Inport  Port=7
  disturbance_torque_y : Inport  Port=8
  disturbance_torque_z : Inport  Port=9
  Constant20 : Constant  Value=Quad_Model  OutDataTypeStr=Bus: Quad_Model_Bus
  Integrator{1..5,100} (6 alike) : Integrator
  MATLAB Function4 : MATLAB Function  TreatAsAtomicUnit=on
  Mux : Mux  Inputs=3
  Mux1 : Mux  Inputs=3
  Mux2 : Mux  Inputs=3
  roll : Outport  VectorParamsAs1DForOutWhenUnconnected=off
  roll_rate : Outport  Port=2  VectorParamsAs1DForOutWhenUnconnected=off
  pitch : Outport  Port=3  VectorParamsAs1DForOutWhenUnconnected=off
  pitch_rate : Outport  Port=4  VectorParamsAs1DForOutWhenUnconnected=off
  yaw : Outport  Port=5  VectorParamsAs1DForOutWhenUnconnected=off
  yaw_rate : Outport  Port=6  VectorParamsAs1DForOutWhenUnconnected=off
  wires:
  Integrator100/1 -> roll_rate/1, Integrator3/1
  Integrator4/1 -> pitch/1
  MATLAB Function4/3(yaw_ddot) -> Integrator2/1
  Integrator3/1 -> roll/1
  Integrator1/1 -> pitch_rate/1, Integrator4/1
  Integrator2/1 -> yaw_rate/1, Integrator5/1
  MATLAB Function4/1(roll_ddot) -> Integrator100/1
  MATLAB Function4/2(pitch_ddot) -> Integrator1/1
  Integrator5/1 -> yaw/1
  disturbance_torque_y/1 -> Mux2/2
  disturbance_torque_z/1 -> Mux2/3
  disturbance_torque_x/1 -> Mux2/1
  Mux2/1 -> MATLAB Function4/3(disturbance_torque)
  yaw_dot/1 -> Mux1/3
  pitch_dot/1 -> Mux1/2
  roll_dot/1 -> Mux1/1
  Mux1/1 -> MATLAB Function4/2(euler_dot)
  torque_y/1 -> Mux/2
  torque_z/1 -> Mux/3
  torque_x/1 -> Mux/1
  Mux/1 -> MATLAB Function4/1(torque)
  Constant20/1 -> MATLAB Function4/4(Quad_Model)

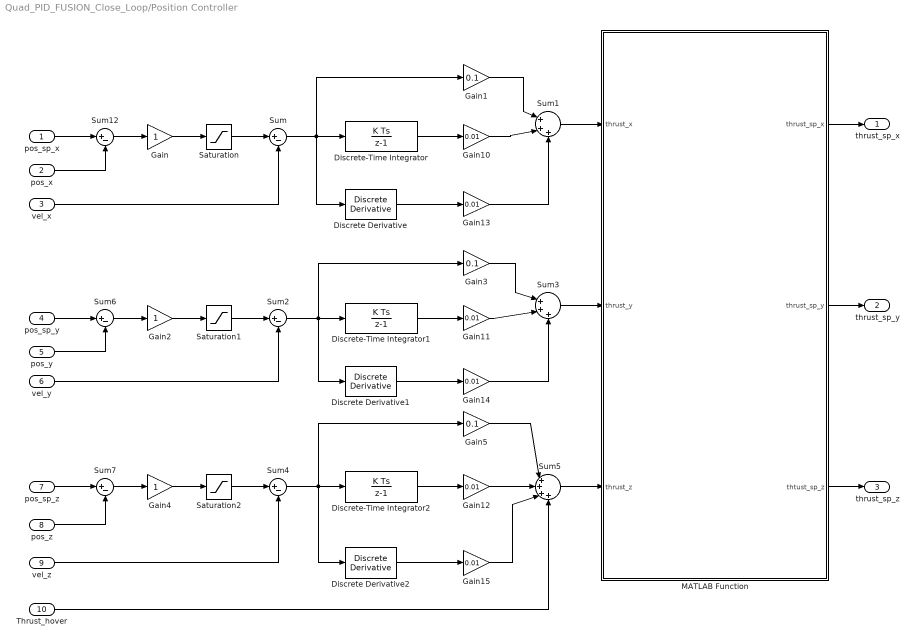
== system Quad_PID_FUSION_Close_Loop/Position Controller ==
  pos_sp_x : Inport
  pos_x : Inport  Port=2
  vel_x : Inport  Port=3
  pos_sp_y : Inport  Port=4
  pos_y : Inport  Port=5
  vel_y : Inport  Port=6
  pos_sp_z : Inport  Port=7
  pos_z : Inport  Port=8
  vel_z : Inport  Port=9
  Thrust_hover : Inport  Port=10
  Discrete Derivative : simulink/Discrete/Discrete Derivative  gainval=1.0  ICPrevScaledInput=0.0  OutMin=[]  OutMax=[]  OutDataType=fixdt(1, 16)  OutScaling=2^-10  DoSatur=off
  Discrete Derivative1 : simulink/Discrete/Discrete Derivative  gainval=1.0  ICPrevScaledInput=0.0  OutMin=[]  OutMax=[]  OutDataType=fixdt(1, 16)  OutScaling=2^-10  DoSatur=off
  Discrete Derivative2 : simulink/Discrete/Discrete Derivative  gainval=1.0  ICPrevScaledInput=0.0  OutMin=[]  OutMax=[]  OutDataType=fixdt(1, 16)  OutScaling=2^-10  DoSatur=off
  Discrete-Time Integrator : DiscreteIntegrator  SampleTime=-1  LimitOutput=on  UpperSaturationLimit=0.9  LowerSaturationLimit=-0.9  ICPrevOutput=DiscIntNeverNeededParam  ICPrevScaledInput=DiscIntNeverNeededParam
  Discrete-Time Integrator1 : DiscreteIntegrator  SampleTime=-1  LimitOutput=on  UpperSaturationLimit=0.9  LowerSaturationLimit=-0.9  ICPrevOutput=DiscIntNeverNeededParam  ICPrevScaledInput=DiscIntNeverNeededParam
  Discrete-Time Integrator2 : DiscreteIntegrator  SampleTime=-1  LimitOutput=on  UpperSaturationLimit=0.9  LowerSaturationLimit=-0.9  ICPrevOutput=DiscIntNeverNeededParam  ICPrevScaledInput=DiscIntNeverNeededParam
  Gain : Gain
  Gain1 : Gain  Gain=0.1
  Gain{10..15} (6 alike) : Gain  Gain=0.01
  Gain2 : Gain
  Gain3 : Gain  Gain=0.1
  Gain4 : Gain
  Gain5 : Gain  Gain=0.1
  MATLAB Function : MATLAB Function  TreatAsAtomicUnit=on
  Saturation : Saturate  UpperLimit=5  LowerLimit=-5
  Saturation1 : Saturate  UpperLimit=5  LowerLimit=-5
  Saturation2 : Saturate  UpperLimit=2  LowerLimit=-2
  Sum{,2,4,6..7,12} (6 alike) : Sum  Inputs=|+-
  Sum1 : Sum  Inputs=|+++
  Sum3 : Sum  Inputs=|+++
  Sum5 : Sum  Inputs=|++++
  thrust_sp_x : Outport  VectorParamsAs1DForOutWhenUnconnected=off
  thrust_sp_y : Outport  Port=2  VectorParamsAs1DForOutWhenUnconnected=off
  thrust_sp_z : Outport  Port=3  VectorParamsAs1DForOutWhenUnconnected=off
  wires:
  Gain4/1 -> Saturation2/1
  Saturation1/1 -> Sum2/1
  MATLAB Function/1(thrust_sp_x) -> thrust_sp_x/1
  vel_x/1 -> Sum/2
  Gain/1 -> Saturation/1
  Gain11/1 -> Sum3/2
  Sum2/1 -> Discrete-Time Integrator1/1, Discrete Derivative1/1, Gain3/1
  Gain3/1 -> Sum3/1
  Sum4/1 -> Discrete-Time Integrator2/1, Discrete Derivative2/1, Gain5/1
  vel_z/1 -> Sum4/2
  Gain2/1 -> Saturation1/1
  Sum5/1 -> MATLAB Function/3(thrust_z)
  Discrete Derivative2/1 -> Gain15/1
  Saturation2/1 -> Sum4/1
  Discrete-Time Integrator/1 -> Gain10/1
  MATLAB Function/2(thrust_sp_y) -> thrust_sp_y/1
  MATLAB Function/3(thtust_sp_z) -> thrust_sp_z/1
  Saturation/1 -> Sum/1
  Gain1/1 -> Sum1/1
  Sum1/1 -> MATLAB Function/1(thrust_x)
  Gain13/1 -> Sum1/3
  Sum/1 -> Discrete-Time Integrator/1, Discrete Derivative/1, Gain1/1
  Discrete Derivative1/1 -> Gain14/1
  Discrete Derivative/1 -> Gain13/1
  Discrete-Time Integrator2/1 -> Gain12/1
  Discrete-Time Integrator1/1 -> Gain11/1
  Thrust_hover/1 -> Sum5/4
  Gain5/1 -> Sum5/1
  Sum3/1 -> MATLAB Function/2(thrust_y)
  Gain12/1 -> Sum5/2
  Gain15/1 -> Sum5/3
  Gain14/1 -> Sum3/3
  vel_y/1 -> Sum2/2
  pos_sp_x/1 -> Sum12/1
  Sum12/1 -> Gain/1
  pos_x/1 -> Sum12/2
  pos_sp_z/1 -> Sum7/1
  Sum7/1 -> Gain4/1
  pos_z/1 -> Sum7/2
  pos_y/1 -> Sum6/2
  Sum6/1 -> Gain2/1
  pos_sp_y/1 -> Sum6/1
  Gain10/1 -> Sum1/2

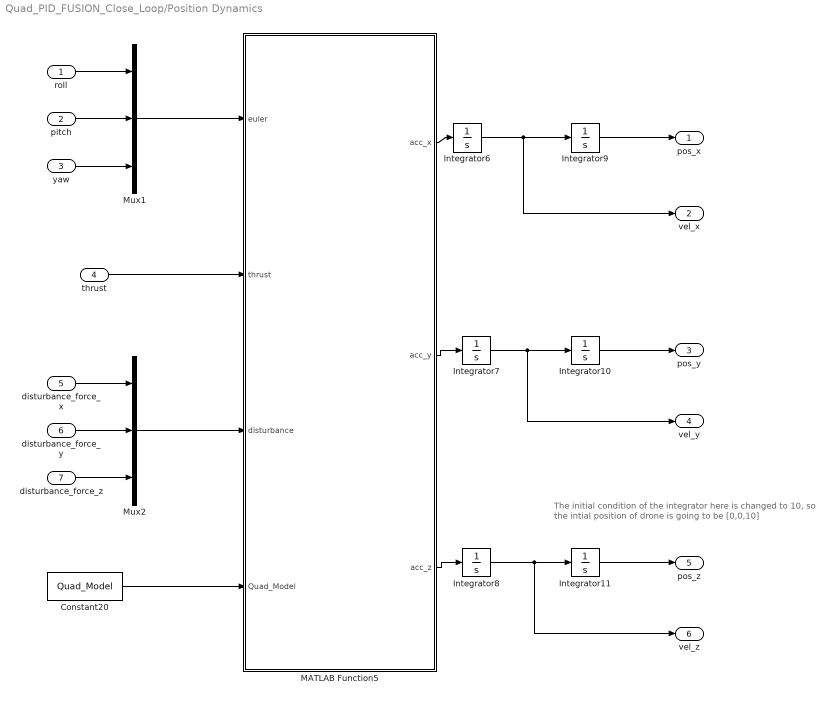
== system Quad_PID_FUSION_Close_Loop/Position Dynamics ==
  note: The initial condition of the integrator here is changed to 10,
      | so the intial position of drone is going to be [0,0,10]
  roll : Inport
  pitch : Inport  Port=2
  yaw : Inport  Port=3
  thrust : Inport  Port=4
  disturbance_force_x : Inport  Port=5
  disturbance_force_y : Inport  Port=6
  disturbance_force_z : Inport  Port=7
  Constant20 : Constant  Value=Quad_Model  OutDataTypeStr=Bus: Quad_Model_Bus
  Integrator{6..10} (5 alike) : Integrator
  Integrator11 : Integrator  InitialCondition=10
  MATLAB Function5 : MATLAB Function  TreatAsAtomicUnit=on
  Mux1 : Mux  Inputs=3
  Mux2 : Mux  Inputs=3
  pos_x : Outport  VectorParamsAs1DForOutWhenUnconnected=off
  vel_x : Outport  Port=2  VectorParamsAs1DForOutWhenUnconnected=off
  pos_y : Outport  Port=3  VectorParamsAs1DForOutWhenUnconnected=off
  vel_y : Outport  Port=4  VectorParamsAs1DForOutWhenUnconnected=off
  pos_z : Outport  Port=5  VectorParamsAs1DForOutWhenUnconnected=off
  vel_z : Outport  Port=6  VectorParamsAs1DForOutWhenUnconnected=off
  wires:
  Integrator7/1 -> vel_y/1, Integrator10/1
  MATLAB Function5/1(acc_x) -> Integrator6/1
  MATLAB Function5/3(acc_z) -> Integrator8/1
  Integrator6/1 -> vel_x/1, Integrator9/1
  MATLAB Function5/2(acc_y) -> Integrator7/1
  thrust/1 -> MATLAB Function5/2(thrust)
  Integrator8/1 -> vel_z/1, Integrator11/1
  Integrator9/1 -> pos_x/1
  Integrator10/1 -> pos_y/1
  Integrator11/1 -> pos_z/1
  roll/1 -> Mux1/1
  pitch/1 -> Mux1/2
  Mux1/1 -> MATLAB Function5/1(euler)
  yaw/1 -> Mux1/3
  disturbance_force_x/1 -> Mux2/1
  disturbance_force_z/1 -> Mux2/3
  Mux2/1 -> MATLAB Function5/3(disturbance)
  disturbance_force_y/1 -> Mux2/2
  Constant20/1 -> MATLAB Function5/4(Quad_Model)

== matlab function Quad_PID_FUSION_Close_Loop/thrust_to_motor_speed ==
  data: w_1 output; torque_x input; torque_y input; w_2 output; torque_z input; thrust input; w_3 output; w_4 output
function [w_1, w_2, w_3, w_4] = thrust_to_motor_speed(torque_x, torque_y, torque_z, thrust)


w_1 = 0;
w_2 = 0;
w_3 = 0;
w_4 = 0;

d  = 0.2;
cT_est = 1.239e-5;
cM_est = 1.982e-7;


M4 = [-sqrt(2)/2*d*cT_est,sqrt(2)/2*d*cT_est,sqrt(2)/2*d*cT_est,-sqrt(2)/2*d*cT_est;
       sqrt(2)/2*d*cT_est,-sqrt(2)/2*d*cT_est,sqrt(2)/2*d*cT_est,-sqrt(2)/2*d*cT_est;
       cM_est,cM_est,-cM_est,-cM_est;
       cT_est,cT_est,cT_est,cT_est;];

w =  M4 \ [torque_x;torque_y;torque_z;thrust];

% w_1 = sqrt(w(1));
% w_2 = sqrt(w(2));
% w_3 = sqrt(w(3));
% w_4 = sqrt(w(4));

w_1 = sqrt(max([0,w(1)]));
w_2 = sqrt(max([0,w(2)]));
w_3 = sqrt(max([0,w(3)]));
w_4 = sqrt(max([0,w(4)]));


end

== matlab function Quad_PID_FUSION_Close_Loop/GPS ==
  settings: updateMethod=DISCRETE
  data: local_pos_gps output; pos_x input; pos_y input; pos_z input; vel_x input; vel_gps output; vel_y input; vel_z input
function [local_pos_gps, vel_gps] = GPS2LLA2GPS(pos_x, pos_y, pos_z, vel_x, vel_y, vel_z)

%GPS
gpsFs = 1;
% GPS = gpsSensor('UpdateRate', gpsFs);
GPS = gpsSensor('ReferenceFrame','NED','SampleRate',gpsFs);
GPS.HorizontalPositionAccuracy = 1;
GPS.VerticalPositionAccuracy = 1;
GPS.VelocityAccuracy = 0.1;
% [lla_pos,lla_vel] = GPS([pos(1),pos(2),pos(3)], [vel(1),vel(2),vel(3)]);
[lla_pos,lla_vel] = GPS([pos_x,pos_y,pos_z], [vel_x,vel_y,vel_z]);
lla0 = [0, 0, 0];
method = 'flat';
local_pos_gps = lla2ned(lla_pos,lla0,method);
vel_gps = lla_vel;

== matlab function Quad_PID_FUSION_Close_Loop/Attitude Dynamics/MATLAB Function4 ==
  data: roll_ddot output; torque input; euler_dot input; pitch_ddot output; yaw_ddot output; disturbance_torque input; Quad_Model input
function [roll_ddot, pitch_ddot, yaw_ddot] = Attitude_Dynamics(torque,euler_dot,disturbance_torque, Quad_Model)


roll_ddot  = 0;
pitch_ddot = 0;
yaw_ddot = 0;

% Quad_Model.Ixx = 0.016;
% Quad_Model.Iyy = 0.016;
% Quad_Model.Izz = 0.0274;
% Quad_Model.Im = 3.789*1e-6;  

roll_ddot  =  disturbance_torque(1) + euler_dot(2) *  euler_dot(3) * (Quad_Model.Iyy - Quad_Model.Izz) / Quad_Model.Ixx - Quad_Model.Im *  euler_dot(2) * 10 + torque(1) / Quad_Model.Ixx;
pitch_ddot =  disturbance_torque(2) + euler_dot(1) *  euler_dot(3) * (Quad_Model.Izz - Quad_Model.Ixx) / Quad_Model.Iyy + Quad_Model.Im *  euler_dot(1) * 10 + torque(2) / Quad_Model.Iyy;
yaw_ddot   =  disturbance_torque(3) + euler_dot(1) *  euler_dot(2) * (Quad_Model.Ixx - Quad_Model.Iyy) / Quad_Model.Izz + torque(3) / Quad_Model.Izz;



end

== matlab function Quad_PID_FUSION_Close_Loop/Position Dynamics/MATLAB Function5 ==
  data: acc_x output; euler input; thrust input; disturbance input; acc_y output; acc_z output; Quad_Model input
function [acc_x,acc_y,acc_z] = Position_Dynamics(euler,thrust,disturbance, Quad_Model)
% Quad_Model.mass = 1;
% Quad_Model.g = 9.8;

acc_x = 0;
acc_y = 0;
acc_z = 0;

acc_x = disturbance(1) + (cos(euler(1)) * sin(euler(2)) * cos(euler(3)) + sin(euler(1)) * sin(euler(3))) * thrust / Quad_Model.mass;
acc_y = disturbance(2) + (cos(euler(1)) * sin(euler(2)) * sin(euler(3)) - sin(euler(1)) * cos(euler(3))) * thrust / Quad_Model.mass;
acc_z = disturbance(3) - Quad_Model.g + cos(euler(1)) * cos(euler(2)) * thrust / Quad_Model.mass;    

end

== matlab function Quad_PID_FUSION_Close_Loop/motor_speed_to_throttle  ==
  data: w_1 input; throttle_1 output; w_2 input; w_3 input; w_4 input; throttle_2 output; throttle_3 output; throttle_4 output
function [throttle_1, throttle_2, throttle_3, throttle_4] = motor_speed_to_throttle(w_1, w_2, w_3, w_4)
    %%注意转速单位 rad/s or rpm 转/分   
    k_est = 718.07;
    d_est = 88.448;
    
    throttle_1 = (w_1 - d_est)/k_est;
    throttle_2 = (w_2 - d_est)/k_est;
    throttle_3 = (w_3 - d_est)/k_est;
    throttle_4 = (w_4 - d_est)/k_est;
end

== matlab function Quad_PID_FUSION_Close_Loop/throttle_to_motor_speed ==
  data: throttle_1 input; w_1 output; throttle_2 input; throttle_3 input; throttle_4 input; w_2 output; w_3 output; w_4 output
function [w_1, w_2, w_3, w_4] = throttle_tomotor_speed(throttle_1, throttle_2, throttle_3, throttle_4)
    k = 718.07;
    d = 88.448;
    
    w_1 = k * throttle_1 + d;
    w_2 = k * throttle_2 + d;
    w_3 = k * throttle_3 + d;
    w_4 = k * throttle_4 + d;
end

== matlab function Quad_PID_FUSION_Close_Loop/motor_speed_to_thrust ==
  data: torque_x output; w_1 input; w_2 input; torque_y output; w_3 input; w_4 input; torque_z output; thrust output
function [torque_x, torque_y, torque_z, thrust] = thrust_to_motor_speed(w_1, w_2, w_3, w_4)

d  = 0.2;
cT = 1.239e-5;
cM = 1.982e-7;


M4 = [-sqrt(2)/2*d*cT,sqrt(2)/2*d*cT,sqrt(2)/2*d*cT,-sqrt(2)/2*d*cT;
       sqrt(2)/2*d*cT,-sqrt(2)/2*d*cT,sqrt(2)/2*d*cT,-sqrt(2)/2*d*cT;
       cM,cM,-cM,-cM;
       cT,cT,cT,cT;];
   
u = M4 * [w_1^2 ;w_2^2 ;w_3^2 ;w_4^2];  

torque_x = u(1);
torque_y = u(2);
torque_z = u(3);
thrust   = u(4);


end

== matlab function Quad_PID_FUSION_Close_Loop/GPSIMUFUSION ==
  settings: updateMethod=DISCRETE
  data: pos_x input; pos_y input; pos_z input; vel_x input; vel_y input; vel_z input; fusedPos output; fusedVel output; acc_x input; acc_y input; acc_z input; roll input; pitch input; yaw input; roll_rate input; pitch_rate input; yaw_rate input; gps_position_noise input; gps_velocity_noise input; fusedOrientEuler output; fusedAngularVel output; imu_acc_noise input; imu_gyro_noise input; imu_mag_noise input; imu_counter output
function [fusedPos,  fusedVel, fusedOrientEuler, fusedAngularVel, imu_counter] = GPSIMUFUSION(pos_x, pos_y, pos_z, vel_x, vel_y, vel_z, acc_x, acc_y, acc_z, roll, pitch, yaw, roll_rate, pitch_rate, yaw_rate, gps_position_noise, gps_velocity_noise, imu_acc_noise, imu_gyro_noise, imu_mag_noise)

% Persistent variable to count IMU updates
persistent imuUpdateCounter
if isempty(imuUpdateCounter)
    imuUpdateCounter = 0;
end

% Increment IMU update counter
imuUpdateCounter = imuUpdateCounter + 1;


% Euler2Quat
eul = [roll, pitch, yaw];
sequence = 'XYZ';
quat = eul2quat(eul,sequence);

imuFs = 100;
gpsFs = 10;

% IMU
% IMU = imuSensor('accel-gyro-mag','ReferenceFrame','NED','SampleRate',imuFs,Seed=66);
IMU = imuSensor('accel-gyro-mag','ReferenceFrame','NED','SampleRate', imuFs);
% Accelerometer
IMU.Accelerometer.MeasurementRange =  19.6133;
IMU.Accelerometer.Resolution = 0.0023928;
IMU.Accelerometer.ConstantBias = 0.19;
IMU.Accelerometer.NoiseDensity = 0.0012356;

% Gyroscope
IMU.Gyroscope.MeasurementRange = deg2rad(250);
IMU.Gyroscope.Resolution = deg2rad(0.0625);
IMU.Gyroscope.ConstantBias = deg2rad(0.125);
IMU.Gyroscope.AxesMisalignment = 1.5;
IMU.Gyroscope.NoiseDensity = deg2rad(0.025);

% Magnetometer
IMU.Magnetometer.MeasurementRange = 1000;
IMU.Magnetometer.Resolution = 0.1;
IMU.Magnetometer.ConstantBias = 100;
IMU.Magnetometer.NoiseDensity = 0.3/ sqrt(50);

% GPS
GPS = gpsSensor('ReferenceFrame','NED','SampleRate',gpsFs);
% GPS.DecayFactor = 0.5;
GPS.HorizontalPositionAccuracy = 1.0;
GPS.VerticalPositionAccuracy = 0.5;
GPS.VelocityAccuracy = 0.05;
% GPS.HorizontalPositionAccuracy = 0;
% GPS.VerticalPositionAccuracy = 0;
% GPS.VelocityAccuracy = 0;
GPS.ReferenceLocation = [0, 0, 0];

% Add noise for GPS
pos_x = pos_x + gps_position_noise(1);
pos_y = pos_y + gps_position_noise(2);
pos_z = pos_z + gps_position_noise(3);
vel_x = vel_x + gps_velocity_noise(1);
vel_y = vel_y + gps_velocity_noise(2);
vel_z = vel_z + gps_velocity_noise(3);

% Filter
fusionfilt = insfilterMARG;
fusionfilt.IMUSampleRate = imuFs;
fusionfilt.ReferenceLocation = [0, 0, 0];

% Measurement noises
Rmag = 0.0862; % Magnetometer measurement noise
Rvel = 0.1; % GPS Velocity measurement noise
Rpos = 1; % GPS Position measurement noise

% Process noises
fusionfilt.AccelerometerBiasNoise =  0.010716; 
fusionfilt.AccelerometerNoise = 9.7785; 
fusionfilt.GyroscopeBiasNoise = 1.3436e-14; 
fusionfilt.GyroscopeNoise =  0.00016528; 
fusionfilt.MagnetometerBiasNoise = 2.189e-11;
fusionfilt.GeomagneticVectorNoise = 7.67e-13;

% Initial error covariance
fusionfilt.StateCovariance = 1e-9*eye(22);
initstate = zeros(22,1);
initstate(1:4) = quat; 
initstate(5:7) = [pos_x, pos_y, pos_z];
initstate(8:10) = [vel_x, vel_y, vel_z];
initstate(11:13) =  IMU.Gyroscope.ConstantBias./imuFs;
initstate(14:16) =  IMU.Accelerometer.ConstantBias./imuFs;
initstate(17:19) =  IMU.MagneticField;
initstate(20:22) = IMU.Magnetometer.ConstantBias;
fusionfilt.State = initstate;


% Get Sensor measurements from GPS and IMU
accs = [acc_x, acc_y, acc_z];
euler_rates = [roll_rate, pitch_rate, yaw_rate];

[accel, gyro, mag] = IMU(accs, euler_rates);

% Add noise for IMU
accel(1) = accel(1) + imu_acc_noise(1);
accel(2) = accel(2) + imu_acc_noise(2);
accel(3) = accel(3) + imu_acc_noise(3);
gyro(1) = gyro(1) + imu_gyro_noise(1);
gyro(2) = gyro(2) + imu_gyro_noise(2);
gyro(3) = gyro(3) + imu_gyro_noise(3);
mag(1) = mag(1) + imu_mag_noise(1);
mag(2) = mag(2) + imu_mag_noise(2);
mag(3) = mag(3) + imu_mag_noise(3);

% Predict
fusionfilt.predict(accel, gyro);

% Fuse GPS
% Check if it's time to fuse GPS data
gpsUpdateCounter = 10;
if imuUpdateCounter >= gpsUpdateCounter % Assuming gpsUpdateCounter is 100 for 1Hz GPS
    [lla_pos,lla_vel] = GPS([pos_x,pos_y,pos_z], [vel_x,vel_y,vel_z]);
    fusionfilt.fusegps(lla_pos, Rpos, lla_vel, Rvel); % Fuse GPS data
    % fusionfilt.fusegps(lla_pos, Rpos);
    imuUpdateCounter = 0; % Reset counter after GPS fusion
end

fusionfilt.fusemag(mag, Rmag);
[fusedPos, fusedOrient] = pose(fusionfilt);
fusedOrientEuler = eulerd(fusedOrient,'XYZ','frame');
fusedOrientEuler = fusedOrientEuler/180 * pi;

state = fusionfilt.State;
fusedVel = state(8:10);
fusedAngularVel = gyro;

imu_counter = imuUpdateCounter;

end

== matlab function Quad_PID_FUSION_Close_Loop/EKF ==
  data: x_hat_ekf input; P input; Y input; x_hat_d_ekf output; input input; P_d output; k output; Quad_Model input
function [x_hat_d_ekf,P_d,k] = EKF(x_hat_ekf, P, Y, input, Quad_Model)

X_hat1=x_hat_ekf(1);
X_hat2=x_hat_ekf(2);
X_hat3=x_hat_ekf(3);
X_hat4=x_hat_ekf(4);
X_hat5=x_hat_ekf(5);
X_hat6=x_hat_ekf(6);


% Quad_Model.Ixx = 0.016;
% Quad_Model.Iyy = 0.016;
% Quad_Model.Izz = 0.0274;
% Quad_Model.Im = 3.789*1e-6;  
% Quad_Model.mass = 1;
M = 1;
Quad_Model.g = 9.8;
a1 = (Quad_Model.Iyy - Quad_Model.Izz) / Quad_Model.Ixx;
a2 = (Quad_Model.Izz - Quad_Model.Ixx) / Quad_Model.Iyy;
a3 = (Quad_Model.Ixx - Quad_Model.Iyy) / Quad_Model.Izz;
b1 = 1/ Quad_Model.Ixx;
b2 = 1/ Quad_Model.Iyy;
b3 = 1/ Quad_Model.Izz;

z_34 = a1*X_hat6- Quad_Model.Im; 
z_35 = a1*X_hat5;
    
z_43 = a2*X_hat6+ Quad_Model.Im; 
z_45 = a2*X_hat4;

z_53 = a3*X_hat5;
z_54 = a3*X_hat4;

z_90 = (-sin(X_hat1)*sin(X_hat2)*cos(X_hat3)+cos(X_hat1)*sin(X_hat3))*(1/M)*input(4);

z_91 = (cos(X_hat1)*cos(X_hat2)*cos(X_hat3))*(1/M)*input(4);
z_92 = (-cos(X_hat1)*sin(X_hat2)*sin(X_hat3)+sin(X_hat1)*cos(X_hat3))*(1/M)*input(4);


z_100 = (-sin(X_hat1)*sin(X_hat2)*sin(X_hat3)-cos(X_hat1)*cos(X_hat3))*(1/M)*input(4);
z_101 = (cos(X_hat1)*cos(X_hat2)*sin(X_hat3))*(1/M)*input(4);
z_102 = (cos(X_hat1)*sin(X_hat2)*cos(X_hat3)+sin(X_hat1)*sin(X_hat3))*(1/M)*input(4);

z_110 = -(1/M)*sin(X_hat1)*cos(X_hat2)*input(4);
z_111 = -(1/M)*cos(X_hat1)*sin(X_hat2)*input(4);

A=[ 0, 0, 0, 1, 0, 0, 0, 0, 0, 0, 0, 0;...
    0, 0, 0, 0, 1, 0, 0, 0, 0, 0, 0, 0;...  
    0, 0, 0, 0, 0, 1, 0, 0, 0, 0, 0, 0;...
    0, 0, 0, 0, z_34, z_35, 0, 0, 0, 0, 0, 0;...
    0, 0, 0, z_43, 0,  z_45, 0, 0, 0, 0, 0, 0;...
    0, 0, 0, z_53, z_54, 0, 0, 0, 0, 0, 0, 0;...                                                                      
    0, 0, 0, 0, 0, 0, 0, 0, 0, 1, 0, 0;...
    0, 0, 0, 0, 0, 0, 0, 0, 0, 0, 1, 0;...
    0, 0, 0, 0, 0, 0, 0, 0, 0, 0, 0, 1;...
    z_90, z_91, z_92, 0, 0, 0, 0, 0, 0, 0, 0, 0;...
    z_100, z_101, z_102, 0, 0, 0, 0, 0, 0, 0, 0, 0;...
    z_110, z_111, 0, 0, 0, 0, 0, 0, 0, 0, 0, 0];

p = 12;
n = 12;
q = .001;
Q = q*eye(n);
Q(1,1)=0;Q(2,2)=0;Q(3,3)=0;Q(7,7)=0;Q(8,8)=0;Q(9,9)=0;
% Q= q*diag([0,0,0,1,1,1,0,0,0,1,1,1]);
r = .001;
R = r*eye(p);

% H=zeros(6,12);H(1,1)=1;H(2,2)=1;H(3,3)=1;H(4,7)=1;H(5,8)=1;H(6,9)=1;
H = eye(12);

K = P*H'*inv(R);
P_d = A*P+P*A'-K*H*P+Q;

x_hat_d_ekf=zeros(12,1);

x_hat_d_ekf(1)= x_hat_ekf(4)+K(1,:)*(Y-H*x_hat_ekf);

x_hat_d_ekf(2)= x_hat_ekf(5)+K(2,:)*(Y-H*x_hat_ekf);

x_hat_d_ekf(3)= x_hat_ekf(6)+K(3,:)*(Y-H*x_hat_ekf);

x_hat_d_ekf(4)  =    x_hat_ekf(5) *  x_hat_ekf(6) * a1 - Quad_Model.Im *  x_hat_ekf(5) * Quad_Model.g + input(1) * b1 + K(4,:)*(Y-H*x_hat_ekf);

x_hat_d_ekf(5)  =    x_hat_ekf(4) *  x_hat_ekf(6) * a2 + Quad_Model.Im *  x_hat_ekf(4) * Quad_Model.g + input(2) *b2 +K(5,:)*(Y-H*x_hat_ekf);

x_hat_d_ekf(6)  =    x_hat_ekf(4) *  x_hat_ekf(5) * a3 + input(3) *b3 +K(6,:)*(Y-H*x_hat_ekf);
        
  
x_hat_d_ekf(7)= x_hat_ekf(10) +K(7,:)*(Y-H*x_hat_ekf);

x_hat_d_ekf(8)= x_hat_ekf(11) +K(8,:)*(Y-H*x_hat_ekf);

x_hat_d_ekf(9)= x_hat_ekf(12) +K(9,:)*(Y-H*x_hat_ekf);


x_hat_d_ekf(10)  =  (cos(x_hat_ekf(1)) * sin(x_hat_ekf(2)) * cos(x_hat_ekf(3)) + sin(x_hat_ekf(1)) * sin(x_hat_ekf(3))) * input(4) / Quad_Model.mass +K(10,:)*(Y-H*x_hat_ekf);

x_hat_d_ekf(11)  =  (cos(x_hat_ekf(1)) * sin(x_hat_ekf(2)) * sin(x_hat_ekf(3)) - sin(x_hat_ekf(1)) * cos(x_hat_ekf(3))) * input(4) / Quad_Model.mass +K(11,:)*(Y-H*x_hat_ekf);

x_hat_d_ekf(12)  =  - Quad_Model.g + cos(x_hat_ekf(1)) * cos(x_hat_ekf(2)) * input(4) / Quad_Model.mass +K(12,:)*(Y-H*x_hat_ekf);    

k=norm(K);
